simulink model "MCA_v2"  (Simulink 8.2)
settings: Solver=ode15s  StartTime=0.0  StopTime=end_time  RelTol=1e-3
values from neighbouring files (symbols this model uses):
  k0 = 1.25    [MCA_model_v2_SDO_init_Normals.m]    (also in MCA_model_v2_SDO_init_Spiking_Selection.m; MCA_model_v2_SDO_init_Trauma.m; MCA_model_v2_coeff_determination_ALL.m = MCADataValues(:,1); MCA_model_v2_coeff_determination_Normals.m = MCADataValues(:,2))
  k1 = 3.75    [MCA_model_v2_SDO_init_Normals.m]    (also in MCA_model_v2_SDO_init_Spiking_Selection.m; MCA_model_v2_SDO_init_Trauma.m; MCA_model_v2_coeff_determination_ALL.m = MCADataValues(:,2); MCA_model_v2_coeff_determination_Normals.m = MCADataValues(:,3))
  k2 = 2.5    [MCA_model_v2_SDO_init_Normals.m]    (also in MCA_model_v2_SDO_init_Spiking_Selection.m; MCA_model_v2_SDO_init_Trauma.m; MCA_model_v2_coeff_determination_ALL.m = MCADataValues(:,3); MCA_model_v2_coeff_determination_Normals.m = MCADataValues(:,4))
  kd = 1.5    [MCA_model_v2_SDO_init_Normals.m]    (also in MCA_model_v2_SDO_init_Spiking_Selection.m; MCA_model_v2_SDO_init_Trauma.m; MCA_model_v2_clustering_ALL.m = [kd; MCADataValues(:,5)]; MCA_model_v2_clustering_Trauma.m = MCADataValues(:,5))
  kn = 12    [MCA_model_v2_SDO_init_Normals.m]    (also in MCA_model_v2_SDO_init_Spiking_Selection.m; MCA_model_v2_SDO_init_Trauma.m; MCA_model_v2_coeff_determination_ALL.m = MCADataValues(:,4); MCA_model_v2_coeff_determination_Normals.m = MCADataValues(:,5))
  TF_init = 5    [MCA_model_v2_SDO_init_Normals.m]    (also in MCA_model_v2_SDO_init_Spiking_Selection.m; MCA_model_v2_SDO_init_Trauma.m)
settings Model: Creator=amenezes  LastModifiedBy=amenezes

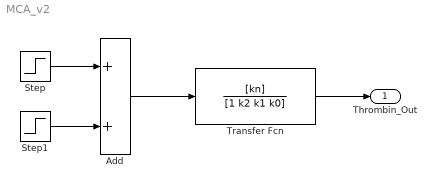
== system MCA_v2 ==
  Add : Sum
  Step : Step  Time=kd  After=TF_init  SampleTime=0
  Step1 : Step  Time=kd+0.01  After=-TF_init  SampleTime=0
  Transfer Fcn : TransferFcn  Numerator=[kn]  Denominator=[1 k2 k1 k0]
  Thrombin_Out : Outport
  wires:
  Transfer Fcn/1 -> Thrombin_Out/1
  Step/1 -> Add/1
  Add/1 -> Transfer Fcn/1
  Step1/1 -> Add/2
